simulink model "Hiv_skogestadsparametere"  (R2022a)
settings: Solver=VariableStepAuto  StartTime=0.0  StopTime=15  RelTol=1e-3
values from neighbouring files (symbols this model uses):
  A_topp = 0.286615    [Modell_verdier.m]
  C_D = 1.28    [Modell_verdier.m]
  g = 9.81    [Modell_verdier.m]
  masse = 22.49    [Modell_verdier.m]
  tetthet_vann = 1000    [Modell_verdier.m]
libraries: spsFirstOrderFilterLib x4
settings Model: Creator=andre  LastModifiedBy=andre

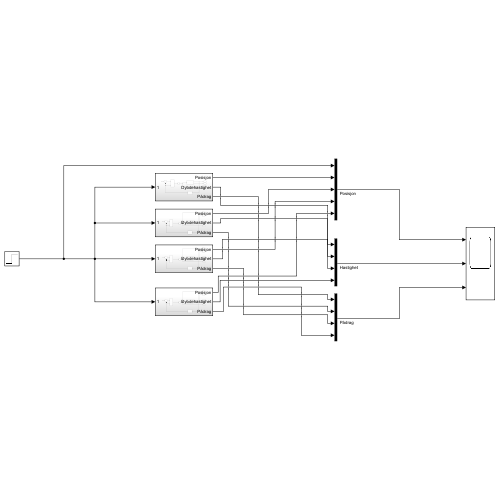
[thumbnail: Simulink's stored preview of the top-level diagram]
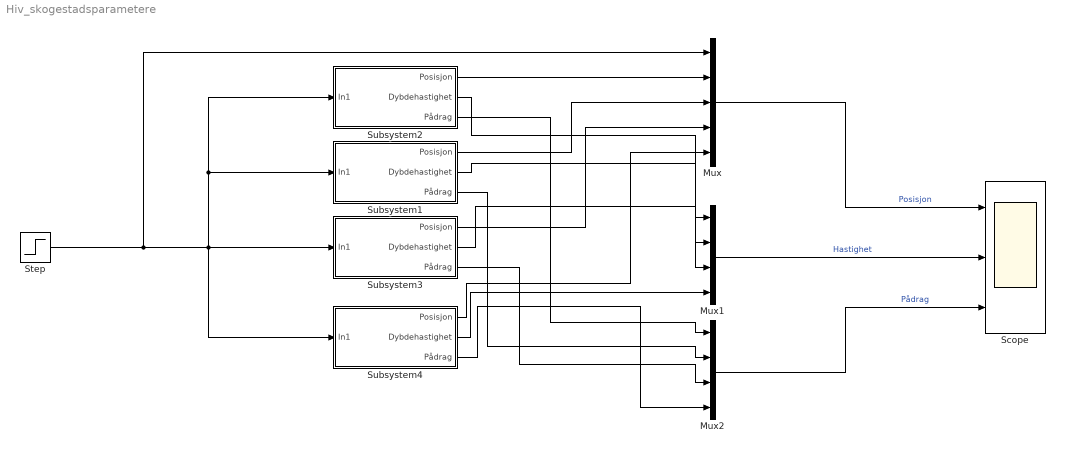
== system Hiv_skogestadsparametere ==
  Mux : Mux  Inputs=5
  Mux1 : Mux
  Mux2 : Mux
  Scope : Scope  NumInputPorts=3
  Step : Step  After=0.4  SampleTime=0
  Subsystem1 : Subsystem
  Subsystem2 : Subsystem
  Subsystem3 : Subsystem
  Subsystem4 : Subsystem
  wires:
  Step/1 -> Mux/1, Subsystem4/1(In1), Subsystem3/1(In1), Subsystem1/1(In1), Subsystem2/1(In1)
  Subsystem2/1(Posisjon) -> Mux/2
  Subsystem1/1(Posisjon) -> Mux/3
  Subsystem3/1(Posisjon) -> Mux/4
  Subsystem4/1(Posisjon) -> Mux/5
  Subsystem4/3(Pådrag) -> Mux2/4
  Subsystem3/3(Pådrag) -> Mux2/3
  Subsystem1/3(Pådrag) -> Mux2/2
  Subsystem2/3(Pådrag) -> Mux2/1
  Subsystem2/2(Dybdehastighet) -> Mux1/1
  Subsystem1/2(Dybdehastighet) -> Mux1/2
  Subsystem3/2(Dybdehastighet) -> Mux1/3
  Subsystem4/2(Dybdehastighet) -> Mux1/4
  Mux/1 -> Scope/1  "Posisjon"
  Mux1/1 -> Scope/2  "Hastighet"
  Mux2/1 -> Scope/3  "Pådrag"

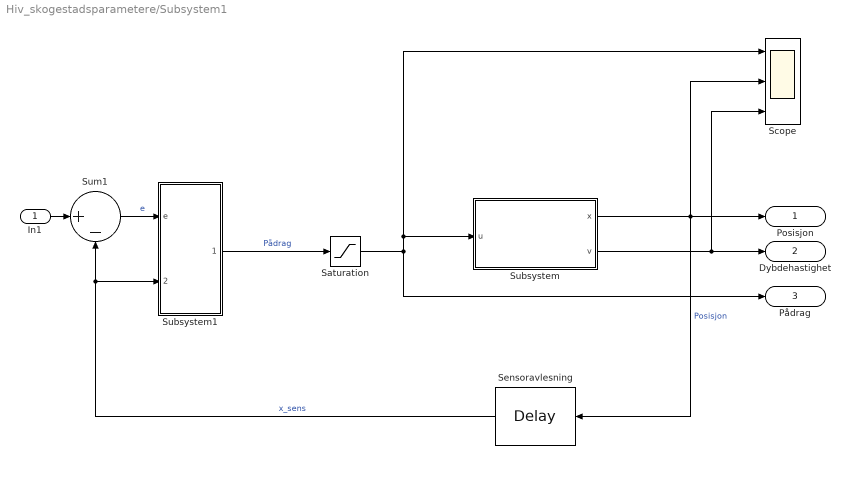
== system Hiv_skogestadsparametere/Subsystem1 ==
  In1 : Inport
  Saturation : Saturate  UpperLimit=2.8  LowerLimit=-2.8
  Scope : Scope  NumInputPorts=3
  Sensoravlesning : TransportDelay  DelayTime=0.2
  Subsystem : Subsystem
  Subsystem1 : Subsystem
  Sum1 : Sum  Inputs=|+-
  Posisjon : Outport
  Dybdehastighet : Outport  Port=2
  Pådrag : Outport  Port=3
  wires:
  Saturation/1 -> Pådrag/1, Scope/1, Subsystem/1(u)
  Subsystem/1(x) -> Posisjon/1, Sensoravlesning/1, Scope/2  "Posisjon"
  Sensoravlesning/1 -> Sum1/2, Subsystem1/2(y_sensor)  "x_sens"
  Subsystem/2(v) -> Dybdehastighet/1, Scope/3
  Subsystem1/1(Pådrag) -> Saturation/1  "Pådrag"
  In1/1 -> Sum1/1
  Sum1/1 -> Subsystem1/1(e)  "e"

== system Hiv_skogestadsparametere/Subsystem2 ==
  In1 : Inport
  Saturation : Saturate  UpperLimit=2.8  LowerLimit=-2.8
  Sensoravlesning : TransportDelay  DelayTime=0.2
  Subsystem : Subsystem
  Subsystem1 : Subsystem
  Sum1 : Sum  Inputs=|+-
  Posisjon : Outport
  Dybdehastighet : Outport  Port=2
  Pådrag : Outport  Port=3
  wires:
  Saturation/1 -> Pådrag/1, Subsystem/1(u)
  Subsystem/1(x) -> Posisjon/1, Sensoravlesning/1  "Posisjon"
  Sensoravlesning/1 -> Sum1/2, Subsystem1/2(y_sensor)  "Signal med forsinkelse"
  Subsystem/2(v) -> Dybdehastighet/1
  Subsystem1/1(Pådrag) -> Saturation/1  "Pådrag"
  In1/1 -> Sum1/1
  Sum1/1 -> Subsystem1/1(e)  "e"

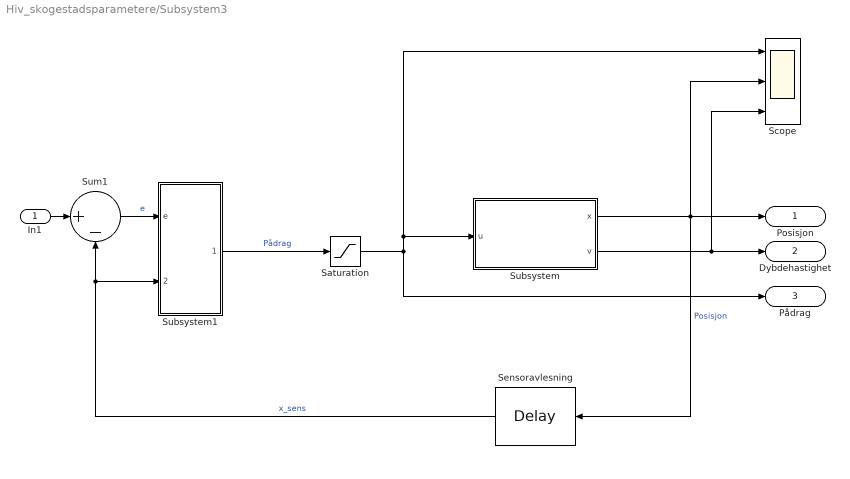
== system Hiv_skogestadsparametere/Subsystem3 ==
  In1 : Inport
  Saturation : Saturate  UpperLimit=2.8  LowerLimit=-2.8
  Scope : Scope  NumInputPorts=3
  Sensoravlesning : TransportDelay  DelayTime=0.2
  Subsystem : Subsystem
  Subsystem1 : Subsystem
  Sum1 : Sum  Inputs=|+-
  Posisjon : Outport
  Dybdehastighet : Outport  Port=2
  Pådrag : Outport  Port=3
  wires:
  Saturation/1 -> Pådrag/1, Scope/1, Subsystem/1(u)
  Subsystem/1(x) -> Posisjon/1, Sensoravlesning/1, Scope/2  "Posisjon"
  Sensoravlesning/1 -> Sum1/2, Subsystem1/2(y_sensor)  "x_sens"
  Subsystem/2(v) -> Dybdehastighet/1, Scope/3
  Subsystem1/1(Pådrag) -> Saturation/1  "Pådrag"
  In1/1 -> Sum1/1
  Sum1/1 -> Subsystem1/1(e)  "e"

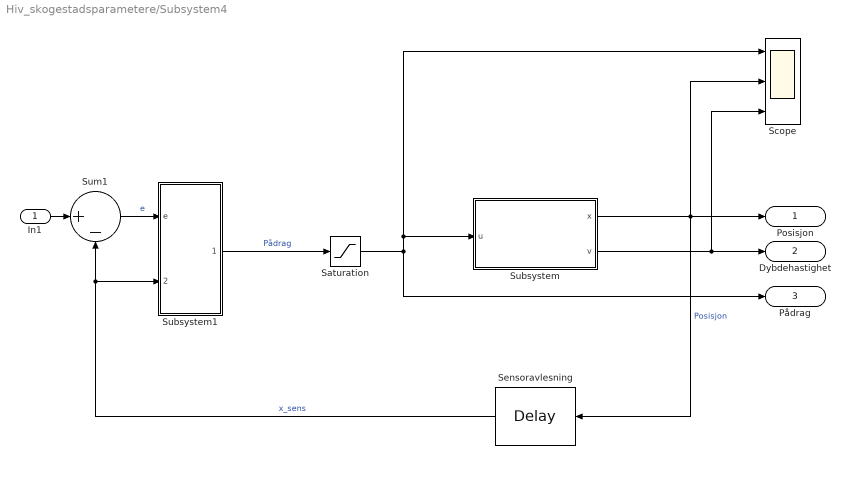
== system Hiv_skogestadsparametere/Subsystem4 ==
  In1 : Inport
  Saturation : Saturate  UpperLimit=2.8  LowerLimit=-2.8
  Scope : Scope  NumInputPorts=3
  Sensoravlesning : TransportDelay  DelayTime=0.2
  Subsystem : Subsystem
  Subsystem1 : Subsystem
  Sum1 : Sum  Inputs=|+-
  Posisjon : Outport
  Dybdehastighet : Outport  Port=2
  Pådrag : Outport  Port=3
  wires:
  Saturation/1 -> Pådrag/1, Scope/1, Subsystem/1(u)
  Subsystem/1(x) -> Posisjon/1, Sensoravlesning/1, Scope/2  "Posisjon"
  Sensoravlesning/1 -> Sum1/2, Subsystem1/2(y_sensor)  "x_sens"
  Subsystem/2(v) -> Dybdehastighet/1, Scope/3
  Subsystem1/1(Pådrag) -> Saturation/1  "Pådrag"
  In1/1 -> Sum1/1
  Sum1/1 -> Subsystem1/1(e)  "e"

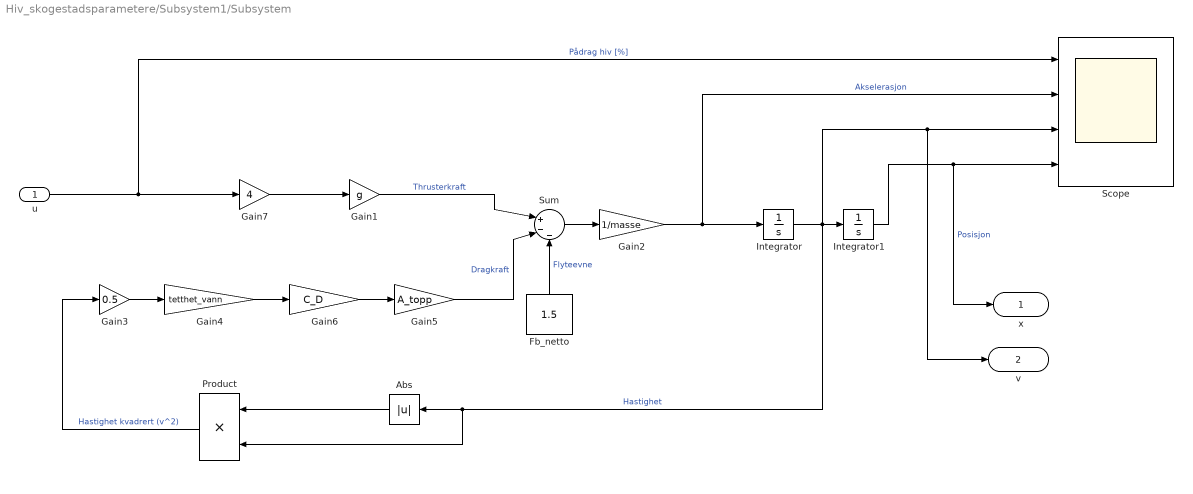
== system Hiv_skogestadsparametere/Subsystem1/Subsystem ==
  u : Inport
  Abs : Abs  SaturateOnIntegerOverflow=off
  Fb_netto : Constant  Value=1.5
  Gain1 : Gain  Gain=g
  Gain2 : Gain  Gain=1/masse
  Gain3 : Gain  Gain=0.5
  Gain4 : Gain  Gain=tetthet_vann
  Gain5 : Gain  Gain=A_topp
  Gain6 : Gain  Gain=C_D
  Gain7 : Gain  Gain=4
  Integrator : Integrator  InitialCondition=0.05
  Integrator1 : Integrator
  Product : Product
  Scope : Scope  NumInputPorts=4
  Sum : Sum  Inputs=|+--
  x : Outport
  v : Outport  Port=2
  wires:
  Gain6/1 -> Gain5/1
  Integrator1/1 -> x/1, Scope/4  "Posisjon"
  Gain5/1 -> Sum/2  "Dragkraft"
  Gain2/1 -> Integrator/1, Scope/2  "Akselerasjon"
  Gain1/1 -> Sum/1  "Thrusterkraft"
  Gain4/1 -> Gain6/1
  Gain3/1 -> Gain4/1
  Fb_netto/1 -> Sum/3  "Flyteevne"
  Integrator/1 -> Integrator1/1, Product/2, Abs/1, v/1, Scope/3  "Hastighet"
  Product/1 -> Gain3/1  "Hastighet kvadrert (v^2)"
  u/1 -> Gain7/1, Scope/1  "Pådrag hiv [%]"
  Abs/1 -> Product/1
  Sum/1 -> Gain2/1
  Gain7/1 -> Gain1/1

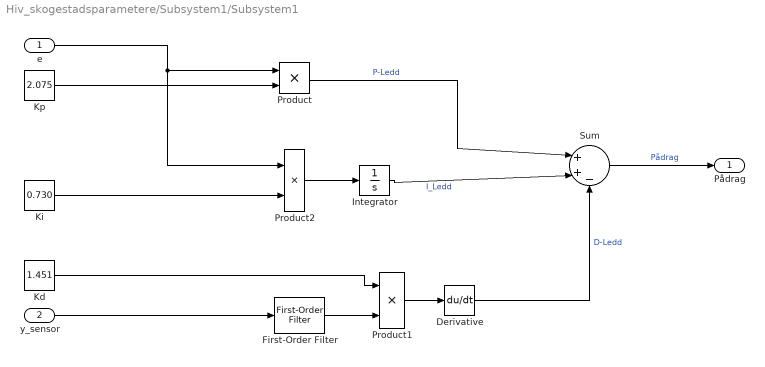
== system Hiv_skogestadsparametere/Subsystem1/Subsystem1 ==
  e : Inport
  y_sensor : Inport  Port=2
  Derivative : Derivative
  First-Order Filter : spsFirstOrderFilterLib/First-Order Filter  FilterType=Lowpass  Tc=(1.451)*0.05  Ts=0  Initialize=on  Vac_Init=[0, 0, 60]  Vdc_Init=0  PlotResponse=off  FreqRange="[0,  200,  1]"
  Integrator : Integrator  LimitOutput=on  UpperSaturationLimit=0.3  LowerSaturationLimit=-0.3
  Kd : Constant  Value=1.451
  Ki : Constant  Value=0.730
  Kp : Constant  Value=2.075
  Product : Product
  Product1 : Product
  Product2 : Product
  Sum : Sum  Inputs=|++-
  Pådrag : Outport
  wires:
  Product2/1 -> Integrator/1
  Kp/1 -> Product/2
  Product/1 -> Sum/1  "P-Ledd"
  y_sensor/1 -> First-Order Filter/1
  Kd/1 -> Product1/1
  e/1 -> Product/1, Product2/1
  Ki/1 -> Product2/2
  First-Order Filter/1 -> Product1/2
  Integrator/1 -> Sum/2  "I_Ledd"
  Sum/1 -> Pådrag/1  "Pådrag"
  Product1/1 -> Derivative/1
  Derivative/1 -> Sum/3  "D-Ledd"

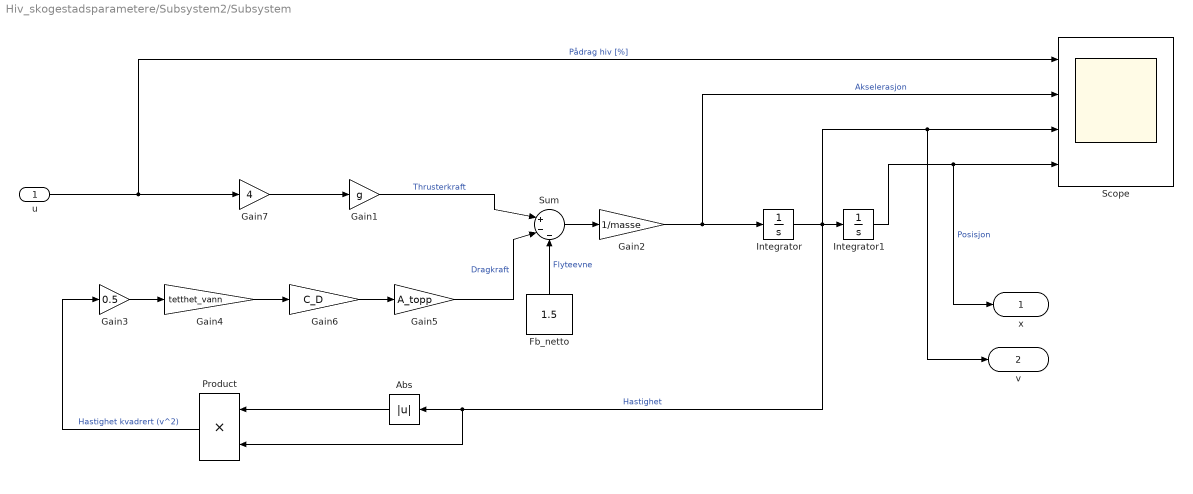
== system Hiv_skogestadsparametere/Subsystem2/Subsystem ==
  u : Inport
  Abs : Abs  SaturateOnIntegerOverflow=off
  Fb_netto : Constant  Value=1.5
  Gain1 : Gain  Gain=g
  Gain2 : Gain  Gain=1/masse
  Gain3 : Gain  Gain=0.5
  Gain4 : Gain  Gain=tetthet_vann
  Gain5 : Gain  Gain=A_topp
  Gain6 : Gain  Gain=C_D
  Gain7 : Gain  Gain=4
  Integrator : Integrator  InitialCondition=0.01
  Integrator1 : Integrator
  Product : Product
  Scope : Scope  NumInputPorts=4
  Sum : Sum  Inputs=|+--
  x : Outport
  v : Outport  Port=2
  wires:
  Gain6/1 -> Gain5/1
  Integrator1/1 -> x/1, Scope/4  "Posisjon"
  Gain5/1 -> Sum/2  "Dragkraft"
  Gain2/1 -> Integrator/1, Scope/2  "Akselerasjon"
  Gain1/1 -> Sum/1  "Thrusterkraft"
  Gain4/1 -> Gain6/1
  Gain3/1 -> Gain4/1
  Fb_netto/1 -> Sum/3  "Flyteevne"
  Integrator/1 -> Integrator1/1, Product/2, Abs/1, v/1, Scope/3  "Hastighet"
  Product/1 -> Gain3/1  "Hastighet kvadrert (v^2)"
  u/1 -> Gain7/1, Scope/1  "Pådrag hiv [%]"
  Abs/1 -> Product/1
  Sum/1 -> Gain2/1
  Gain7/1 -> Gain1/1

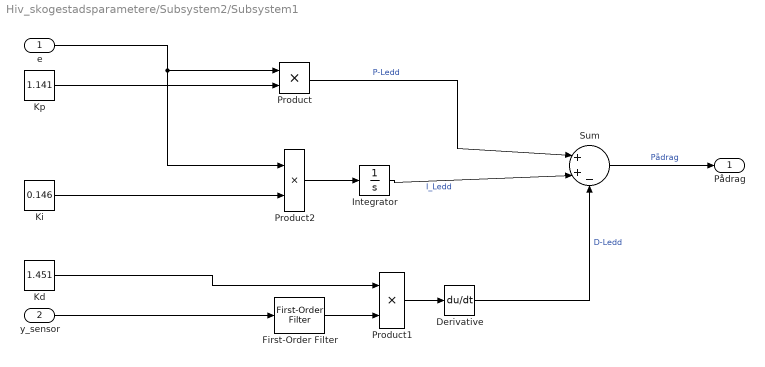
== system Hiv_skogestadsparametere/Subsystem2/Subsystem1 ==
  e : Inport
  y_sensor : Inport  Port=2
  Derivative : Derivative
  First-Order Filter : spsFirstOrderFilterLib/First-Order Filter  FilterType=Lowpass  Tc=(1.5/3.8)*0.05  Ts=0  Initialize=on  Vac_Init=[0, 0, 60]  Vdc_Init=0  PlotResponse=off  FreqRange="[0,  200,  1]"
  Integrator : Integrator  LimitOutput=on  UpperSaturationLimit=0.3  LowerSaturationLimit=-0.3
  Kd : Constant  Value=1.451
  Ki : Constant  Value=0.146
  Kp : Constant  Value=1.141
  Product : Product
  Product1 : Product
  Product2 : Product
  Sum : Sum  Inputs=|++-
  Pådrag : Outport
  wires:
  Product2/1 -> Integrator/1
  Kp/1 -> Product/2
  Product/1 -> Sum/1  "P-Ledd"
  y_sensor/1 -> First-Order Filter/1
  Kd/1 -> Product1/1
  e/1 -> Product/1, Product2/1
  Ki/1 -> Product2/2
  First-Order Filter/1 -> Product1/2
  Integrator/1 -> Sum/2  "I_Ledd"
  Sum/1 -> Pådrag/1  "Pådrag"
  Product1/1 -> Derivative/1
  Derivative/1 -> Sum/3  "D-Ledd"

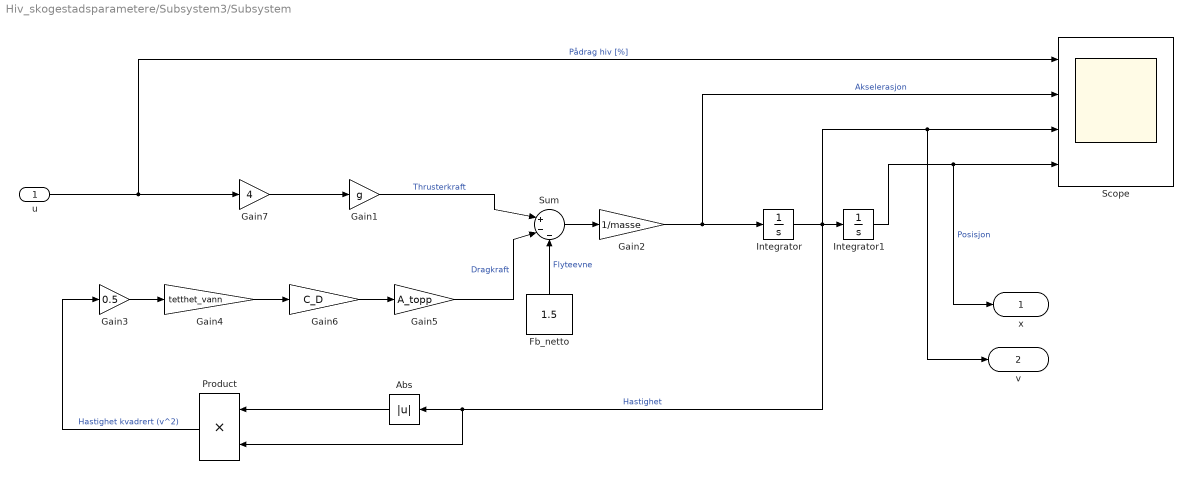
== system Hiv_skogestadsparametere/Subsystem3/Subsystem ==
  u : Inport
  Abs : Abs  SaturateOnIntegerOverflow=off
  Fb_netto : Constant  Value=1.5
  Gain1 : Gain  Gain=g
  Gain2 : Gain  Gain=1/masse
  Gain3 : Gain  Gain=0.5
  Gain4 : Gain  Gain=tetthet_vann
  Gain5 : Gain  Gain=A_topp
  Gain6 : Gain  Gain=C_D
  Gain7 : Gain  Gain=4
  Integrator : Integrator  InitialCondition=0.1
  Integrator1 : Integrator
  Product : Product
  Scope : Scope  NumInputPorts=4
  Sum : Sum  Inputs=|+--
  x : Outport
  v : Outport  Port=2
  wires:
  Gain6/1 -> Gain5/1
  Integrator1/1 -> x/1, Scope/4  "Posisjon"
  Gain5/1 -> Sum/2  "Dragkraft"
  Gain2/1 -> Integrator/1, Scope/2  "Akselerasjon"
  Gain1/1 -> Sum/1  "Thrusterkraft"
  Gain4/1 -> Gain6/1
  Gain3/1 -> Gain4/1
  Fb_netto/1 -> Sum/3  "Flyteevne"
  Integrator/1 -> Integrator1/1, Product/2, Abs/1, v/1, Scope/3  "Hastighet"
  Product/1 -> Gain3/1  "Hastighet kvadrert (v^2)"
  u/1 -> Gain7/1, Scope/1  "Pådrag hiv [%]"
  Abs/1 -> Product/1
  Sum/1 -> Gain2/1
  Gain7/1 -> Gain1/1

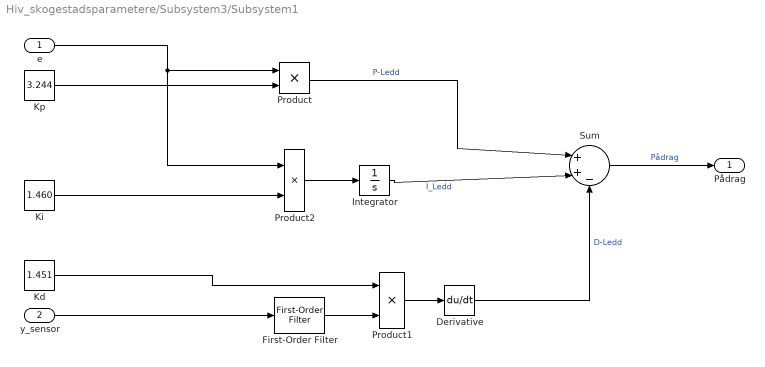
== system Hiv_skogestadsparametere/Subsystem3/Subsystem1 ==
  e : Inport
  y_sensor : Inport  Port=2
  Derivative : Derivative
  First-Order Filter : spsFirstOrderFilterLib/First-Order Filter  FilterType=Lowpass  Tc=(1.451)*0.05  Ts=0  Initialize=on  Vac_Init=[0, 0, 60]  Vdc_Init=0  PlotResponse=off  FreqRange="[0,  200,  1]"
  Integrator : Integrator  LimitOutput=on  UpperSaturationLimit=0.3  LowerSaturationLimit=-0.3
  Kd : Constant  Value=1.451
  Ki : Constant  Value=1.460
  Kp : Constant  Value=3.244
  Product : Product
  Product1 : Product
  Product2 : Product
  Sum : Sum  Inputs=|++-
  Pådrag : Outport
  wires:
  Product2/1 -> Integrator/1
  Kp/1 -> Product/2
  Product/1 -> Sum/1  "P-Ledd"
  y_sensor/1 -> First-Order Filter/1
  Kd/1 -> Product1/1
  e/1 -> Product/1, Product2/1
  Ki/1 -> Product2/2
  First-Order Filter/1 -> Product1/2
  Integrator/1 -> Sum/2  "I_Ledd"
  Sum/1 -> Pådrag/1  "Pådrag"
  Product1/1 -> Derivative/1
  Derivative/1 -> Sum/3  "D-Ledd"

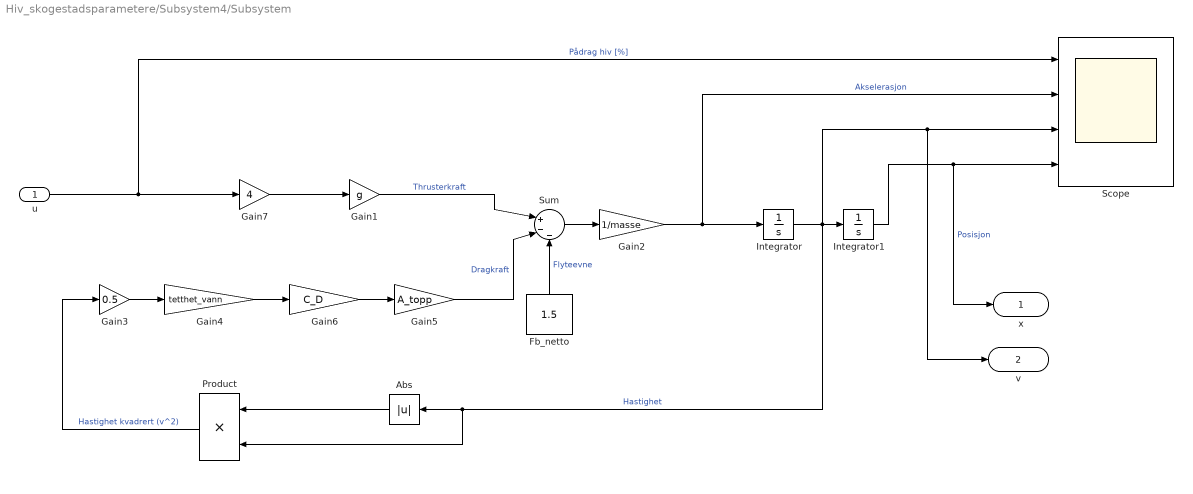
== system Hiv_skogestadsparametere/Subsystem4/Subsystem ==
  u : Inport
  Abs : Abs  SaturateOnIntegerOverflow=off
  Fb_netto : Constant  Value=1.5
  Gain1 : Gain  Gain=g
  Gain2 : Gain  Gain=1/masse
  Gain3 : Gain  Gain=0.5
  Gain4 : Gain  Gain=tetthet_vann
  Gain5 : Gain  Gain=A_topp
  Gain6 : Gain  Gain=C_D
  Gain7 : Gain  Gain=4
  Integrator : Integrator  InitialCondition=0.5
  Integrator1 : Integrator
  Product : Product
  Scope : Scope  NumInputPorts=4
  Sum : Sum  Inputs=|+--
  x : Outport
  v : Outport  Port=2
  wires:
  Gain6/1 -> Gain5/1
  Integrator1/1 -> x/1, Scope/4  "Posisjon"
  Gain5/1 -> Sum/2  "Dragkraft"
  Gain2/1 -> Integrator/1, Scope/2  "Akselerasjon"
  Gain1/1 -> Sum/1  "Thrusterkraft"
  Gain4/1 -> Gain6/1
  Gain3/1 -> Gain4/1
  Fb_netto/1 -> Sum/3  "Flyteevne"
  Integrator/1 -> Integrator1/1, Product/2, Abs/1, v/1, Scope/3  "Hastighet"
  Product/1 -> Gain3/1  "Hastighet kvadrert (v^2)"
  u/1 -> Gain7/1, Scope/1  "Pådrag hiv [%]"
  Abs/1 -> Product/1
  Sum/1 -> Gain2/1
  Gain7/1 -> Gain1/1

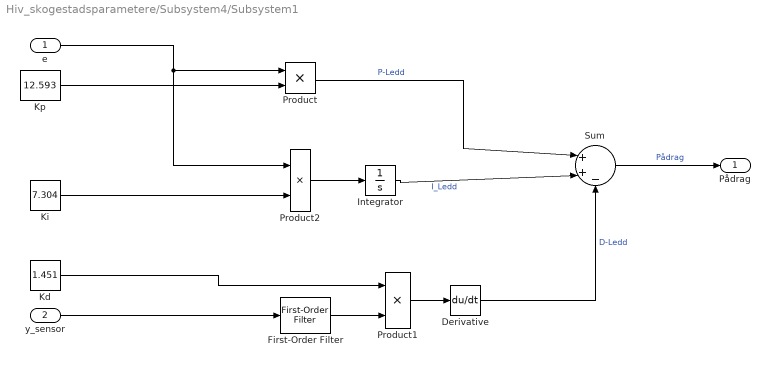
== system Hiv_skogestadsparametere/Subsystem4/Subsystem1 ==
  e : Inport
  y_sensor : Inport  Port=2
  Derivative : Derivative
  First-Order Filter : spsFirstOrderFilterLib/First-Order Filter  FilterType=Lowpass  Tc=(1.451)*0.05  Ts=0  Initialize=on  Vac_Init=[0, 0, 60]  Vdc_Init=0  PlotResponse=off  FreqRange="[0,  200,  1]"
  Integrator : Integrator  LimitOutput=on  UpperSaturationLimit=0.3  LowerSaturationLimit=-0.3
  Kd : Constant  Value=1.451
  Ki : Constant  Value=7.304
  Kp : Constant  Value=12.593
  Product : Product
  Product1 : Product
  Product2 : Product
  Sum : Sum  Inputs=|++-
  Pådrag : Outport
  wires:
  Product2/1 -> Integrator/1
  Kp/1 -> Product/2
  Product/1 -> Sum/1  "P-Ledd"
  y_sensor/1 -> First-Order Filter/1
  Kd/1 -> Product1/1
  e/1 -> Product/1, Product2/1
  Ki/1 -> Product2/2
  First-Order Filter/1 -> Product1/2
  Integrator/1 -> Sum/2  "I_Ledd"
  Sum/1 -> Pådrag/1  "Pådrag"
  Product1/1 -> Derivative/1
  Derivative/1 -> Sum/3  "D-Ledd"
